simulink model "spi_demo"  (Simulink 7.3)
settings: Solver=ode3  SolverMode=SingleTasking  StartTime=0.0  StopTime=10.0  RelTol=1e-3
PreLoadFcn:
  | waijung.modelPreload; % Required for working with Waijung Blockset. Do not remove.
undefined symbols (not defined in the file): LQFP48, STM32F072CB
libraries: stm32f0_device_config_lib x1
CloseFcn:
  | waijung.modelClose; % Required for working with Waijung Blockset. Do not remove.
settings Model: Creator=Krisada  LastModifiedBy=Krisada
settings OptimizationCC: OptimizeModelRefInitCode=on  LifeSpan=1
settings HardwareCC: ProdEndianess=LittleEndian  ProdHWDeviceType=ARM Compatible->Cortex - M0  TargetEndianess=LittleEndian  TargetHWDeviceType=ARM Compatible->Cortex - M0
settings RTWCC: SystemTargetFile=stm32f0.tlc  GenerateMakefile=off  TemplateMakefile=ert_default_tmf  Description=STM32F0 Target  ProcessScript=stm32f0_make_rtw_hook
settings CodeAppCC: IgnoreCustomStorageClasses=off
settings STFCustomTargetCC: ModelReferenceCompliant=off  CombineOutputUpdateFcns=on  ERTCustomFileBanners=on  SupportContinuousTime=off  SupportNonInlinedSFcns=off  SystemTargetFile=stm32f0.tlc
settings ERTTargetCC: MultiwordLength=2048  ModelReferenceCompliant=off  ParMdlRefBuildCompliant=off  CompOptLevelCompliant=off  ERTFirstTimeCompliant=off  ModelStepFunctionPrototypeControlCompliant=off  CPPClassGenCompliant=off  InlinedParameterPlacement=NonHierarchical  ERTSrcFileBannerTemplate=stm32f0_code_template.cgt  ERTHdrFileBannerTemplate=stm32f0_code_template.cgt  ERTDataSrcFileTemplate=stm32f0_code_template.cgt  ERTDataHdrFileTemplate=stm32f0_code_template.cgt  ERTCustomFileTemplate=stm32f0_file_process.tlc

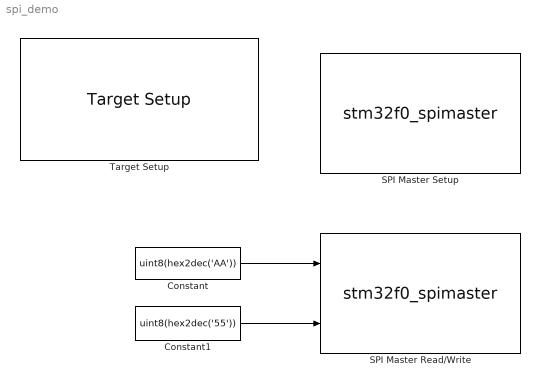
== system spi_demo ==
  Constant : Constant  Value=uint8(hex2dec('AA'))  OutDataType=fixdt(1, 16)  OutScaling=2^0
  Constant1 : Constant  Value=uint8(hex2dec('55'))  OutDataType=fixdt(1, 16)  OutScaling=2^0
  SPI Master Read/Write : S-Function  FunctionName=stm32f0_spimaster  Parameters=mode,configuration,module,datacount,inputtypearray,outputtypearray,confstr,sampletime,sampletimestr,blockid  EnableBusSupport=off  mask(stm32f0_spimaster){configuration=Transaction, module=2, mode=Read/ Write, lastmodule=1, direction=Full-Duplex, dataformat=8bit/ FirstBit_MSB, prescaler=4, cpolcpha=CPOL_Low/ CPHA_1Edge, datacount=2, nssmode=Custom, nsspin=Not used, softnssport=E, softnsspin=0, sckpin=A5, misopin=A6, mosipin=A7, inputtypearray=[2 3 3], outputtypearray=[3 7 3 3], confstr=["SPI_Direction_2Lines_FullDuplex","8b","MSB","Low","1Edge","4","Custom","0","x","x","0","0","x","x","1","A","5","","1","A","6","","1","A","7","","1","0","0","0","0","0","0","0","0","0","0"], sampletime=0.1, sampletimestr=0.1, blockid=SPIMasterReadWrite}
      mask prompts: module "SPI Module:"; lastmodule "Last module:"; dataformat "Data format:"; prescaler "Buad rate prescaler: Pclk/"; cpolcpha "Clock polarity (CPOL)/ Clock phase (CPHA):"; datacount "Data Read/Write count:"; nssmode "Slave/chip select (nSS, nCS) mode"; nsspin "Slave/chip select (nSS, nCS) pin"; softnssport "Slave/chip select port (nSS, nCS)"; softnsspin "Slave/chip select pin (nSS, nCS)"; sckpin "SCLK pin:"; misopin "MISO pin:"; mosipin "MOSI pin:"; inputtypearray "Input type array"; outputtypearray "Output type array"; confstr "Configuration string"; sampletime "Sample time (sec)"; sampletimestr "Compiled sample time (sec) in string"
      mask help:
      | Status:
      |  0 - Success.
      |  Otherwise - Fail.
      mask init:
      | stm32f0_spimaster_callback('init');
      mask Help: web(fullfile(waijungdocroot,'stm32f0_spimaster_readwrite.htm'), '-browser')
      mask StyleString: popup(Setup|Transaction),popup(1|2),popup(Read/ Write|Read|Write),edit,popup(Full-Duplex|Half-Duplex_Tx|Half-Duplex_Rx),popup(8bit/ FirstBit_MSB|8bit/ FirstBit_LSB|16bit/ FirstBit_MSB|16bit/ FirstBit_LSB),popup(2|4|8|16|32|64|128|256),popup(CPOL_Low/ CPHA_1Edge|CPOL_Low/ CPHA_2Edge|CPOL_High/ CPHA_1Edge|CPOL_High/ CPHA_2Edge),edit,popup(Hardware|Software|Custom),popup(Not used|A4|A15),popup(A|B|C|D|E|F|G|H|I),popup(0|1|2|3|4|5|6|7|8|9|10|11|12|13|14|15),popup(Not used|A5|B3),popup(Not used|A6|B4),popup(Not used|A7|B5),edit,edit,edit,edit,edit,edit
      mask CallbackString: stm32f0_spimaster_callback('configuration');|stm32f0_spimaster_callback('module');|stm32f0_spimaster_callback('mode');||stm32f0_spimaster_callback('direction');||||stm32f0_spimaster_callback('datacount');|stm32f0_spimaster_callback('nssmode');|||||||||stm32f0_spimaster_callback('confstr');|stm32f0_spimaster_callback('sampletime');|stm32f0_spimaster_callback('sampletimestr');|stm32f0_spimaster_callback('blockid');
      mask Display: text(0.5, 0.5, 'Module: SPI2 (Master)\nRead/ Write\nTs (sec): 0.1','ver','middle','hor','center');port_label('input', 1,'Wr0 (uint8)');port_label('input', 2,'Wr1 (uint8)');port_label('output', 1,'Status');port_label('output', 2,'Rd0 (uint8)');port_label('output', 3,'Rd1 (uint8)');
  SPI Master Setup : S-Function  FunctionName=stm32f0_spimaster  Parameters=mode,configuration,module,datacount,inputtypearray,outputtypearray,confstr,sampletime,sampletimestr,blockid  EnableBusSupport=off  mask(stm32f0_spimaster){configuration=Setup, module=2, mode=Write, lastmodule=2, direction=Full-Duplex, dataformat=8bit/ FirstBit_MSB, prescaler=4, lastpclk=48000000, baudrate=12000000, cpolcpha=CPOL_Low/ CPHA_1Edge, datacount=0, nssmode=Software, nsspin=Not used, softnssport=B, softnsspin=9, sckpin=B10, misopin=B14, mosipin=B15, nssdelay=0, framedelay=0, inputtypearray=[0], outputtypearray=[0], confstr=["SPI_Direction_2Lines_FullDuplex","8b","MSB","Low","1Edge","4","Soft","0","x","x","0","1","B","9","1","B","10","5","1","B","14","0","1","B","15","0","0","1","0","0","0","0","0","0","0","0","0"], sampletime=-1, sampletimestr=0.1, blockid=SPIMasterSetup}
      mask prompts: module "SPI Module:"; lastmodule "Last module:"; dataformat "Data format:"; prescaler "Buad rate prescaler: Pclk/"; lastpclk "Last PCLK"; baudrate "Baud rate (Hz)"; cpolcpha "Clock polarity (CPOL)/ Clock phase (CPHA):"; datacount "Data Write count:"; nssmode "Slave/chip select (nSS, nCS) mode"; nsspin "Slave/chip select (nSS, nCS) pin"; softnssport "Slave/chip select port (nSS, nCS)"; softnsspin "Slave/chip select pin (nSS, nCS)"; sckpin "SCLK pin:"; misopin "MISO pin:"; mosipin "MOSI pin:"; nssdelay "Slave/chip select (nSS, nCS) delay time (uS)"; framedelay "Data frame delay time (uS)"; inputtypearray "Input type array"; outputtypearray "Output type array"; confstr "Configuration string"; sampletime "Sample time (sec)"; sampletimestr "Compiled sample time (sec) in string"
      mask help:
      | Direction:
      |  - Full-Duplex, use this mode when need to send and receive data at same clock.
      |  - Half-Duplex_Tx, this mode is to transmit data to slave only. Pin MISO (Rx) can be free for other function.
      |  - Half-Duplex_Rx, this mode is to receive data from slave only. Pin MOSIO (Tx) can be free for other function.
      | Data format:
      |   This configuration is depending on the specification of slave device.
      | Baud rate prescaler:
      |  - Use this prescaler to devide from the PCLK for SPI clock.
      |  - This Prescaler value is auto determine corresponding to baudrate setting and selected SPI module.
      | Baud rate (Hz):
      |  - Select baud rate for SPI clock. Please check the maximum clock support for target slave device.
      | Clock polarity and Clock phase:
      |  - This configuration parameter is depending on slave device.
      |  - See waijung help for more description.
      | Slave/chip select mode:
      |  - Hardware, use hardware SPI module for slave select (or chip select) pin.
      |  - Software, this mode allow any available pin for slave select (or chip select) function.
      |  - Custom, SPI block did not control slave select pin. User may use Digital Output block to control by costom.
      mask init:
      | stm32f0_spimaster_callback('init');
      mask Help: web(fullfile(waijungdocroot,'stm32f0_spimaster_setup.htm'), '-browser')
      mask StyleString: popup(Setup|Transaction),popup(1|2),popup(Read/ Write|Read|Write),edit,popup(Full-Duplex|Half-Duplex_Tx|Half-Duplex_Rx),popup(8bit/ FirstBit_MSB|8bit/ FirstBit_LSB|16bit/ FirstBit_MSB|16bit/ FirstBit_LSB),popup(2|4|8|16|32|64|128|256),edit,popup(Not set|12000000|6000000|3000000|1500000|750000|375000|187500),popup(CPOL_Low/ CPHA_1Edge|CPOL_Low/ CPHA_2Edge|CPOL_High/ CPHA_1Edge|CPOL_High/ CPHA_2Edge),edit,popup(Hardware|Software|Custom),popup(Not used|B9|B12|D0),popup(A|B|C|D|E|F|G|H|I),popup(0|1|2|3|4|5|6|7|8|9|10|11|12|13|14|15),popup(Not used|B10|B13|D1),popup(Not used|B14|C2|D3),popup(Not used|B15|C3|D4),edit,edit,edit,edit,edit,edit,edit,edit
      mask CallbackString: stm32f0_spimaster_callback('configuration');|stm32f0_spimaster_callback('module');|stm32f0_spimaster_callback('mode');||stm32f0_spimaster_callback('direction');||||stm32f0_spimaster_callback('baudrate');||stm32f0_spimaster_callback('datacount');|stm32f0_spimaster_callback('nssmode');|||||||||||stm32f0_spimaster_callback('confstr');|stm32f0_spimaster_callback('sampletime');|stm32f0_spimaster_callback('sampletimestr');|stm32f0_spimaster_callback('blockid');
      mask Display: text(0.5, 0.5, 'Module: SPI2 (Master)\nFull-Duplex\nBaudrate: 12000000','ver','middle','hor','center');
  Target Setup : stm32f0_device_config_lib/Target Setup  Priority=100  compiler=GNU ARM  previous_compiler=GNU ARM  mcu=STM32F072CB (LQFP48)  mcustr=STM32F072CB  stdlib=STM32F072  clockconfig=FiO MOTE-ST Default (HSEOSC-8MHz/HCLK-48MHz)  system_stm32f0xx_c_path=F:\trunk\targets\stm32f0_target\stm32f0\utils\STM32F0xx_AN4055\stm32f0_default\hse8mhz_pll_hclk48mhz  showmemoryconfiguration=on  stacksize=0x400  heapsize=0x200  enableautocompiledownload=on  fullchiperase=off  programmerinterface=aMG USB Connect  editctrlstr=on  compilercontrolstr=$(patsubst %, -I%, .) -mcpu=cortex-m0 -mthumb -mabi=aapcs -Wall -O3 -mfloat-abi=soft -ffunction-sections -fdata-sections -fno-strict-aliasing -fno-builtin --short-enums  assemblercontrolstr=$(patsubst %, -I%, .) -mcpu=cortex-m0 -mtune=cortex-m0 -mthumb -Wall -O3 -Wa,-amhls=$(<:.s=.lst) -D__STACK_SIZE=$(STACK_SIZE) -D__HEAP_SIZE=$(HEAP_SIZE)  linkercontrolstr="-T$(LD_SCRIPT) -Wl,-Map=$(MAP),--cref,--no-warn-mismatch -mcpu=cortex-m0 -mthumb  -Wall -O3 -mabi=aapcs -lc -specs=nosys.specs"  runafterdownload=on  execprofile=None  profileruart=3  profilerbaud=500000  profilertxpin=Not used  profilerinitstr=0.1,48000000,4800000,500000,0  manualsetsampletime=off  sampletime=0.1  blockid=TargetSetup  systickreloadvalue=4800000  hseval=8000000  lastprofileruart=3  hclk=48000000  flashorigin=0x8000000  flashlength=128k  ramorigin=0x20000000  ramlength=16k  useextram=off
  wires:
  Constant/1 -> SPI Master Read/Write/1
  Constant1/1 -> SPI Master Read/Write/2
